simulink model "tank_valve_system_nonlin"  (R2017a)
settings: Solver=VariableStepAuto  StartTime=0.0  StopTime=40  MaxStep=0.001  RelTol=1e-3
model workspace (MATLAB code in the model file):
  | A = 1; % Area of tank
  | a = 0.1; % area of hole
  | g = 9.80; % Gravity
  | h0 = 1;   % Operating point
  | z0 = a*sqrt(2*g*h0); % Operating point
  | alpha = a/A * sqrt(2*g/h0);
  | beta = 1/A;
settings Model: Creator=kjartan  LastModifiedBy=kjartan

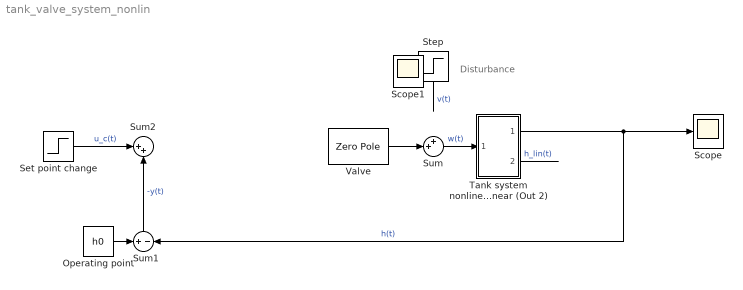
== system tank_valve_system_nonlin ==
  note: Disturbance
  Operating point : Constant  Value=h0
  Scope : Scope
  Set point change : Step  After=0.2  SampleTime=0
  Step : Step  Time=3  After=0.3  SampleTime=0
  Sum : Sum  Inputs=++|
  Sum1 : Sum  Inputs=+|-
  Sum2 : Sum  Inputs=|++
  Tank system nonlinear(Out 1) and linear (Out 2) : Subsystem
  Valve : ZeroPole  Zeros=[]  Poles=[-2 -2]  Gain=[4]
  Scope1 : Scope
  wires:
  Tank system nonlinear(Out 1) and linear (Out 2)/1(Out1) -> Sum1/2, Scope/1  "h(t)"
  Tank system nonlinear(Out 1) and linear (Out 2)/2(Out2) -> ?  "h_lin(t)"
  Sum/1 -> Tank system nonlinear(Out 1) and linear (Out 2)/1(In1)  "w(t)"
  Valve/1 -> Sum/2
  Operating point/1 -> Sum1/1
  Sum1/1 -> Sum2/2  "-y(t)"
  Set point change/1 -> Sum2/1  "u_c(t)"
  ? -> Valve/1  "u(t)"
  Step/1 -> ?  "v(t)"

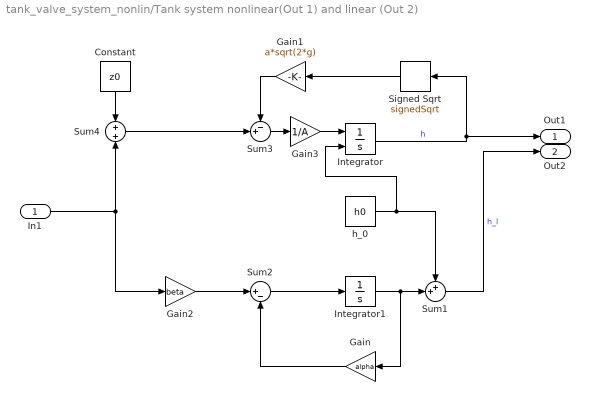
== system tank_valve_system_nonlin/Tank system nonlinear(Out 1) and linear (Out 2) ==
  In1 : Inport
  Constant : Constant  Value=z0
  Gain : Gain  Gain=alpha
  Gain1 : Gain  Gain=a*sqrt(2*g)
  Gain2 : Gain  Gain=beta
  Gain3 : Gain  Gain=1/A
  Integrator : Integrator  InitialConditionSource=external  InitialCondition=h0
  Integrator1 : Integrator
  Signed Sqrt : Sqrt  Operator=signedSqrt  SaturateOnIntegerOverflow=on
  Sum1 : Sum  Inputs=++|
  Sum2 : Sum  Inputs=|+-
  Sum3 : Sum  Inputs=-+|
  Sum4 : Sum  Inputs=+|+
  h_0 : Constant  Value=h0
  Out1 : Outport
  Out2 : Outport  Port=2
  wires:
  Integrator/1 -> Out1/1, Signed Sqrt/1  "h"
  h_0/1 -> Integrator/2, Sum1/1
  Sum1/1 -> Out2/1  "h_l"
  Integrator1/1 -> Gain/1, Sum1/2
  Sum2/1 -> Integrator1/1
  Gain/1 -> Sum2/2
  Signed Sqrt/1 -> Gain1/1
  Sum3/1 -> Gain3/1
  Gain1/1 -> Sum3/1
  In1/1 -> Gain2/1, Sum4/2
  Gain2/1 -> Sum2/1
  Sum4/1 -> Sum3/2
  Constant/1 -> Sum4/1
  Gain3/1 -> Integrator/1
